simulink model "SegwayModel2017"  (R2017b)
settings: Solver=VariableStepAuto  StartTime=0.0  StopTime=10.0  RelTol=1e-3
undefined symbols (not defined in the file): F, g, l, M, m, T, X0
settings Model: Creator=Huynh  LastModifiedBy=Huynh
settings DataIOCC: ReturnWorkspaceOutputs=on
settings OptimizationCC: DefaultParameterBehavior=Inlined  BufferReuse=off
settings DebuggingCC: InitInArrayFormatMsg=none
settings SFSimCC: SimUseLocalCustomCode=on
settings RTWCC: RTWUseLocalCustomCode=on

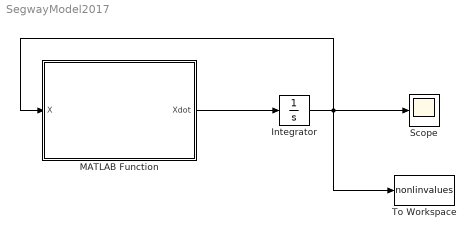
== system SegwayModel2017 ==
  Integrator : Integrator  InitialCondition=X0
  MATLAB Function : MATLAB Function  TreatAsAtomicUnit=on
  Scope : Scope
  To Workspace : ToWorkspace  VariableName=nonlinvalues  SampleTime=-1
  wires:
  MATLAB Function/1(Xdot) -> Integrator/1
  Integrator/1 -> To Workspace/1, MATLAB Function/1(X), Scope/1

== matlab function SegwayModel2017/MATLAB Function ==
  data: X input; Xdot output; m parameter; M parameter; g parameter; l parameter; T parameter; F parameter
function Xdot = nonLinearSegway(X, m, M, g, l, T, F)
x = X(1); xd = X(2); theta = X(3); thetad = X(4);
xdd = (-m*l*thetad^2*sin(theta)+m*g*cos(theta)*sin(theta)+...
    T/l*cos(theta) + F)/(m+M-m*cos(theta)^2);
thetadd = ((M+m)*g*l*sin(theta)- m*m^2*thetad^2*cos(theta)*sin(theta)+...
    (M+m)/m * T+l*F*cos(theta))/((m+M-m*cos(theta)^2)*l^2);
Xdot = [xd; xdd; thetad; thetadd];
end
